simulink model "FYP_Flywheel_Stage2"  (R2024a)
settings: Solver=ode45  StartTime=0.0  StopTime=12  RelTol=1e-3
values from neighbouring files (symbols this model uses):
  B = 1.0e-3    (= 0.001)    [FYP_Flywheel_Stage2_build.m]    (also in FYP_Flywheel_Stage3_DCServo_build.m; FYP_Flywheel_Stage4_v2_StableClosedLoop_build.m; FYP_Flywheel_Stage5_COMPLETE_v2.m)
  J = 0.5    [FYP_Flywheel_Stage1_build.m]    (also in FYP_Flywheel_Stage2_build.m)
  omega0 = 2*pi*n0/60    (= 314.159265359)    [FYP_Flywheel_Stage1_build.m]    (also in FYP_Flywheel_Stage2_build.m; FYP_Flywheel_Stage3_DCServo_build.m; FYP_Flywheel_Stage4_v2_StableClosedLoop_build.m; FYP_Flywheel_Stage5_COMPLETE_v2.m)
  omega_max = 2*pi*n_max/60    (= 356.047167407)    [FYP_Flywheel_Stage2_build.m]    (also in FYP_Flywheel_Stage5_COMPLETE_v2.m = 329.867228627)
  omega_min = 2*pi*n_min/60    (= 293.215314335)    [FYP_Flywheel_Stage2_build.m]    (also in FYP_Flywheel_Stage5_COMPLETE_v2.m = 298.451302091)
  Tc = 0.05    [FYP_Flywheel_Stage2_build.m]    (also in FYP_Flywheel_Stage3_DCServo_build.m; FYP_Flywheel_Stage4_v2_StableClosedLoop_build.m; FYP_Flywheel_Stage5_COMPLETE_v2.m)
settings Model: Creator=cheng  LastModifiedBy=cheng

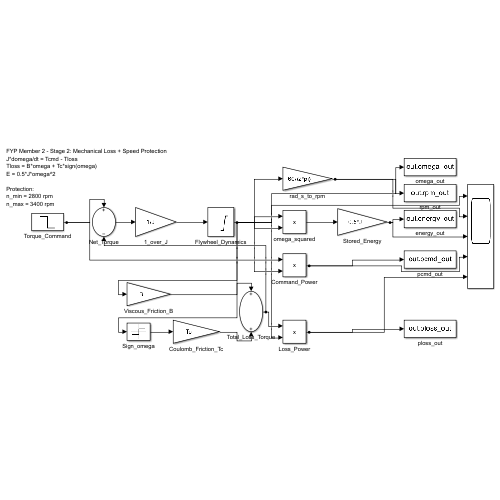
[thumbnail: Simulink's stored preview of the top-level diagram]
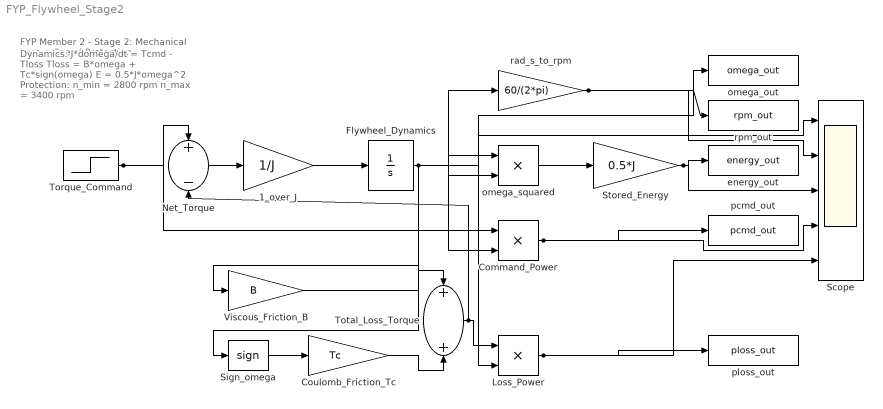
== system FYP_Flywheel_Stage2 ==
  note: FYP Member 2 - Stage 2: Mechanical Loss + Speed Protection
  note: Dynamics:
      | J*domega/dt = Tcmd - Tloss
      | Tloss = B*omega + Tc*sign(omega)
      | E = 0.5*J*omega^2
      |
      | Protection:
      | n_min = 2800 rpm
      | n_max = 3400 rpm
  1_over_J : Gain  Gain=1/J
  Command_Power : Product  Inputs=**
  Coulomb_Friction_Tc : Gain  Gain=Tc
  Flywheel_Dynamics : Integrator  InitialCondition=omega0  LimitOutput=on  UpperSaturationLimit=omega_max  LowerSaturationLimit=omega_min
  Loss_Power : Product  Inputs=**
  Net_Torque : Sum  Inputs=+-
  Scope : Scope  NumInputPorts=5
  Sign_omega : Signum
  Stored_Energy : Gain  Gain=0.5*J
  Torque_Command : Step  Time=4  Before=8  After=-8  SampleTime=0
  Total_Loss_Torque : Sum
  Viscous_Friction_B : Gain  Gain=B
  energy_out : ToWorkspace  VariableName=energy_out  SaveFormat=Timeseries  SampleTime=-1
  omega_out : ToWorkspace  VariableName=omega_out  SaveFormat=Timeseries  SampleTime=-1
  omega_squared : Product  Inputs=**
  pcmd_out : ToWorkspace  VariableName=pcmd_out  SaveFormat=Timeseries  SampleTime=-1
  ploss_out : ToWorkspace  VariableName=ploss_out  SaveFormat=Timeseries  SampleTime=-1
  rad_s_to_rpm : Gain  Gain=60/(2*pi)
  rpm_out : ToWorkspace  VariableName=rpm_out  SaveFormat=Timeseries  SampleTime=-1
  wires:
  Torque_Command/1 -> Net_Torque/1, Command_Power/1
  Net_Torque/1 -> 1_over_J/1
  1_over_J/1 -> Flywheel_Dynamics/1
  Flywheel_Dynamics/1 -> Viscous_Friction_B/1, Sign_omega/1, rad_s_to_rpm/1, omega_squared/1, omega_squared/2, Command_Power/2, Loss_Power/2, omega_out/1, Scope/1
  Viscous_Friction_B/1 -> Total_Loss_Torque/1
  Sign_omega/1 -> Coulomb_Friction_Tc/1
  Coulomb_Friction_Tc/1 -> Total_Loss_Torque/2
  Total_Loss_Torque/1 -> Net_Torque/2, Loss_Power/1
  omega_squared/1 -> Stored_Energy/1
  rad_s_to_rpm/1 -> rpm_out/1, Scope/2
  Stored_Energy/1 -> energy_out/1, Scope/3
  Command_Power/1 -> pcmd_out/1, Scope/4
  Loss_Power/1 -> ploss_out/1, Scope/5
